simulink model "motor"  (R2020a)
settings: Solver=VariableStepAuto  StartTime=0.0  StopTime=10.0  RelTol=1e-3
undefined symbols (not defined in the file or in its folder): b, J, k, L, R
settings Model: Creator=Admin  LastModifiedBy=Admin
settings DataIOCC: ExternalInput=[t,vtg]  LoadExternalInput=on  SaveFormat=Array  ReturnWorkspaceOutputs=off

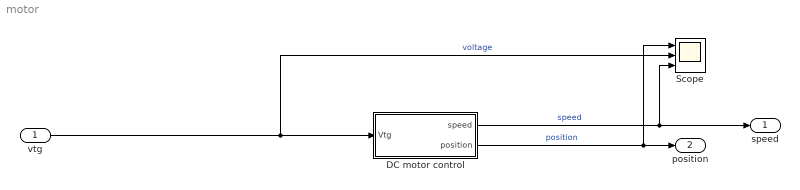
== system motor ==
  vtg : Inport  Interpolate=off
  DC motor control : Subsystem
  Scope : Scope  NumInputPorts=3
  speed : Outport
  position : Outport  Port=2
  wires:
  DC motor control/1(speed) -> Scope/3, speed/1  "speed"
  vtg/1 -> Scope/2, DC motor control/1(Vtg)  "voltage"
  DC motor control/2(position) -> Scope/1, position/1  "position"

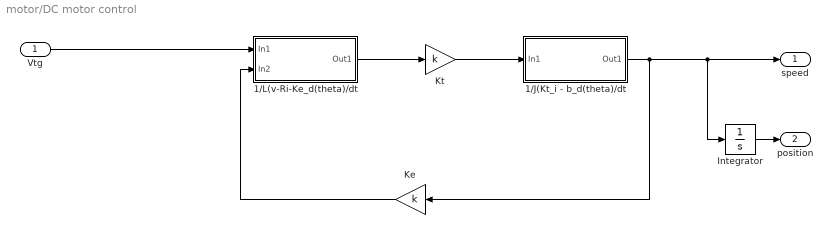
== system motor/DC motor control ==
  Vtg : Inport
  1/J(Kt_i - b_d(theta)/dt : Subsystem
  1/L(v-Ri-Ke_d(theta)/dt : Subsystem
  Integrator : Integrator
  Ke : Gain  Gain=k
  Kt : Gain  Gain=k
  speed : Outport
  position : Outport  Port=2
  wires:
  Ke/1 -> 1/L(v-Ri-Ke_d(theta)/dt/2(In2)
  Vtg/1 -> 1/L(v-Ri-Ke_d(theta)/dt/1(In1)
  Kt/1 -> 1/J(Kt_i - b_d(theta)/dt/1(In1)
  1/L(v-Ri-Ke_d(theta)/dt/1(Out1) -> Kt/1
  1/J(Kt_i - b_d(theta)/dt/1(Out1) -> Integrator/1, speed/1, Ke/1
  Integrator/1 -> position/1

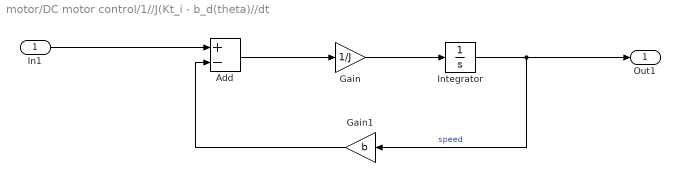
== system motor/DC motor control/1//J(Kt_i - b_d(theta)//dt ==
  In1 : Inport
  Add : Sum  Inputs=+-
  Gain : Gain  Gain=1/J
  Gain1 : Gain  Gain=b
  Integrator : Integrator
  Out1 : Outport
  wires:
  Add/1 -> Gain/1
  Gain/1 -> Integrator/1
  Integrator/1 -> Out1/1, Gain1/1  "speed"
  In1/1 -> Add/1
  Gain1/1 -> Add/2

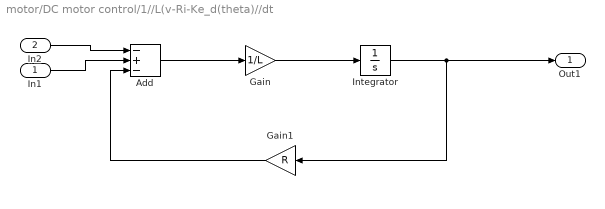
== system motor/DC motor control/1//L(v-Ri-Ke_d(theta)//dt ==
  In1 : Inport
  In2 : Inport  Port=2
  Add : Sum  Inputs=-+-
  Gain : Gain  Gain=1/L
  Gain1 : Gain  Gain=R
  Integrator : Integrator
  Out1 : Outport
  wires:
  In1/1 -> Add/2
  In2/1 -> Add/1
  Add/1 -> Gain/1
  Gain/1 -> Integrator/1
  Integrator/1 -> Gain1/1, Out1/1
  Gain1/1 -> Add/3
